simulink model "pid_parallel_sim"  (R2023a)
settings: Solver=VariableStepAuto  StartTime=0.0  StopTime=0.2  MaxStep=Ts  RelTol=1e-3
values from neighbouring files (symbols this model uses):
  fcutD = fp    (= 300)    [pid_ini_parallel.m]
  fcutrollOff = ff    (= 500)    [pid_ini_parallel.m]
  fp = fp_s    (= 300)    [pid_ini_parallel.m]    (also in pid_ini_series.m)
  g_awr = 1.2    [pid_ini_parallel.m]    (also in pid_ini_series.m = 1)
  Kd = -(Ki_s*fp_s - Ki_s*fz_s - 2*pi*Kp_s*fp_s^2 + 2*pi*Kp_s*fp_s*fz_s)/(4*fp_s^2*fz_s*pi^2)    (= 0.176396728594)    [pid_ini_parallel.m]
  Ki = Ki_s    (= 2356.19449019)    [pid_ini_parallel.m]    (also in pid_ini_series.m)
  Kp = (Ki_s*fp_s - Ki_s*fz_s + 2*pi*Kp_s*fp_s*fz_s)/(2*fp_s*fz_s*pi)    (= 42.5)    [pid_ini_parallel.m]    (also in pid_ini_series.m = 25)
  Ts = 50e-6    (= 5e-05)    [pid_ini_parallel.m]    (also in pid_ini_series.m)
  u_max = 5.5    [pid_ini_parallel.m]    (also in pid_ini_series.m)
  u_min = -u_max    (= -5.5)    [pid_ini_parallel.m]    (also in pid_ini_series.m)
  uMax = u_max    (= 5.5)    [pid_ini_parallel.m]
  uMin = u_min    (= -5.5)    [pid_ini_parallel.m]
libraries: cstblocks x8
settings Model: Creator=Michael Peter  LastModifiedBy=Michael Peter

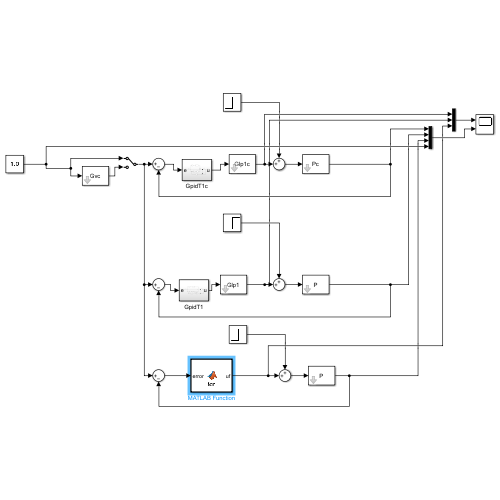
[thumbnail: Simulink's stored preview of the top-level diagram]
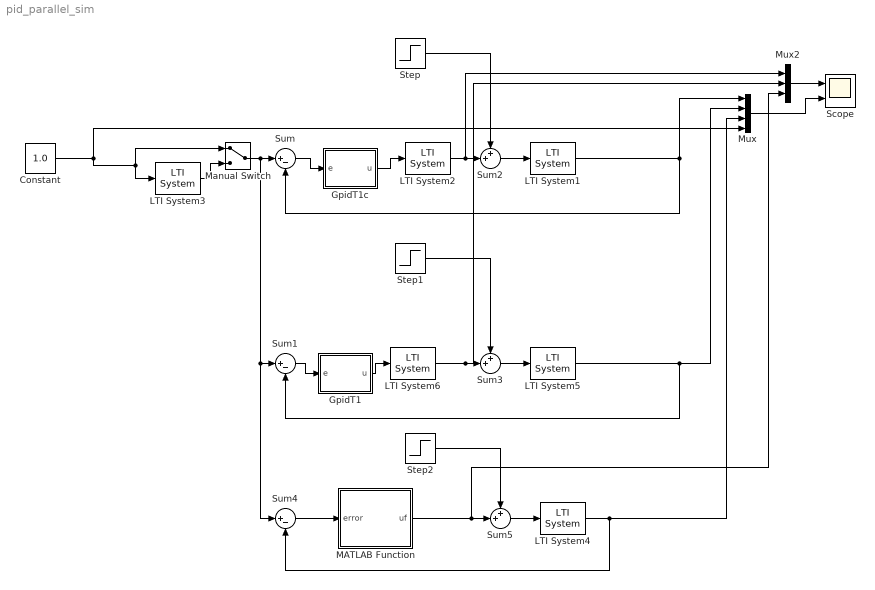
== system pid_parallel_sim ==
  Constant : Constant  Value=1.0
  GpidT1 : Subsystem
  GpidT1c : Subsystem
  LTI System1 : cstblocks/LTI System  sys=Pc  IC=[]
  LTI System2 : cstblocks/LTI System  sys=Glp1c  IC=[]
  LTI System3 : cstblocks/LTI System  sys=Gvc  IC=[]
  LTI System4 : cstblocks/LTI System  sys=P  IC=[]
  LTI System5 : cstblocks/LTI System  sys=P  IC=[]
  LTI System6 : cstblocks/LTI System  sys=Glp1  IC=[]
  MATLAB Function : MATLAB Function  TreatAsAtomicUnit=on
  Manual Switch : ManualSwitch
  Mux : Mux
  Mux2 : Mux  Inputs=3
  Scope : Scope  NumInputPorts=2
  Step : Step  Time=0.12  After=3.5  SampleTime=0
  Step1 : Step  Time=0.12  After=3.5  SampleTime=0
  Step2 : Step  Time=0.12  After=3.5  SampleTime=0
  Sum : Sum  Inputs=|+-
  Sum1 : Sum  Inputs=|+-
  Sum2 : Sum  Inputs=++|
  Sum3 : Sum  Inputs=++|
  Sum4 : Sum  Inputs=|+-
  Sum5 : Sum  Inputs=++|
  wires:
  Sum/1 -> GpidT1c/1(e)
  LTI System1/1 -> Mux/1, Sum/2
  GpidT1c/1(u) -> LTI System2/1
  Sum2/1 -> LTI System1/1
  Mux/1 -> Scope/2
  Step/1 -> Sum2/1
  Manual Switch/1 -> Sum4/1, Sum1/1, Sum/1
  LTI System3/1 -> Manual Switch/2
  Step1/1 -> Sum3/1
  Sum3/1 -> LTI System5/1
  GpidT1/1(u) -> LTI System6/1
  LTI System5/1 -> Mux/2, Sum1/2
  Sum1/1 -> GpidT1/1(e)
  Mux2/1 -> Scope/1
  Sum4/1 -> MATLAB Function/1(error)
  LTI System4/1 -> Mux/3, Sum4/2
  Constant/1 -> Manual Switch/1, LTI System3/1, Mux/4
  Step2/1 -> Sum5/1
  Sum5/1 -> LTI System4/1
  MATLAB Function/1(uf) -> Mux2/3, Sum5/2
  LTI System6/1 -> Mux2/2, Sum3/2
  LTI System2/1 -> Mux2/1, Sum2/2

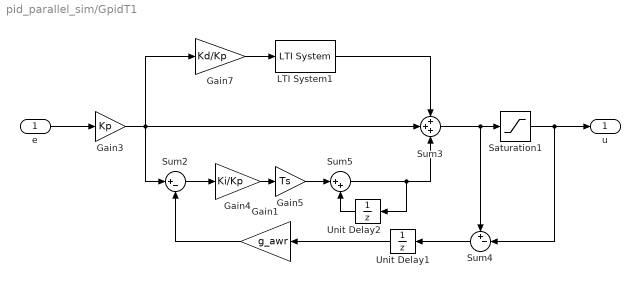
== system pid_parallel_sim/GpidT1 ==
  e : Inport
  Gain1 : Gain  Gain=g_awr
  Gain3 : Gain  Gain=Kp
  Gain4 : Gain  Gain=Ki/Kp
  Gain5 : Gain  Gain=Ts
  Gain7 : Gain  Gain=Kd/Kp
  LTI System1 : cstblocks/LTI System  sys=Gd  IC=[]
  Saturation1 : Saturate  UpperLimit=u_max  LowerLimit=u_min
  Sum2 : Sum  Inputs=|+-
  Sum3 : Sum  Inputs=+++
  Sum4 : Sum  Inputs=+-|
  Sum5 : Sum  Inputs=|++
  Unit Delay1 : UnitDelay  SampleTime=Ts  HasFrameUpgradeWarning=on
  Unit Delay2 : UnitDelay  SampleTime=Ts  HasFrameUpgradeWarning=on
  u : Outport
  wires:
  Gain1/1 -> Sum2/2
  e/1 -> Gain3/1
  Sum5/1 -> Sum3/3, Unit Delay2/1
  Gain5/1 -> Sum5/1
  Gain3/1 -> Gain7/1, Sum3/2, Sum2/1
  Sum2/1 -> Gain4/1
  Gain4/1 -> Gain5/1
  Sum4/1 -> Unit Delay1/1
  Sum3/1 -> Sum4/1, Saturation1/1
  Saturation1/1 -> u/1, Sum4/2
  Unit Delay1/1 -> Gain1/1
  Unit Delay2/1 -> Sum5/2
  Gain7/1 -> LTI System1/1
  LTI System1/1 -> Sum3/1

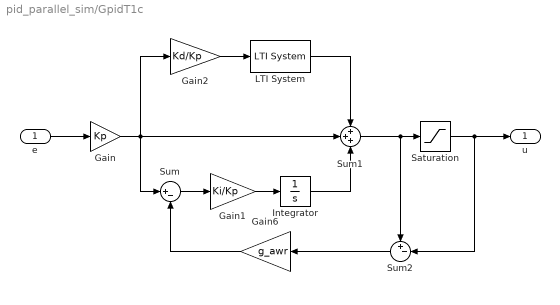
== system pid_parallel_sim/GpidT1c ==
  e : Inport
  Gain : Gain  Gain=Kp
  Gain1 : Gain  Gain=Ki/Kp
  Gain2 : Gain  Gain=Kd/Kp
  Gain6 : Gain  Gain=g_awr
  Integrator : Integrator
  LTI System : cstblocks/LTI System  sys=(2*pi*fp) * tf([1 0], [1 2*pi*fp])  IC=[]
  Saturation : Saturate  UpperLimit=u_max  LowerLimit=u_min
  Sum : Sum  Inputs=|+-
  Sum1 : Sum  Inputs=+++
  Sum2 : Sum  Inputs=+-|
  u : Outport
  wires:
  Saturation/1 -> u/1, Sum2/2
  Sum1/1 -> Sum2/1, Saturation/1
  Gain1/1 -> Integrator/1
  Sum2/1 -> Gain6/1
  Gain/1 -> Sum1/2, Gain2/1, Sum/1
  Sum/1 -> Gain1/1
  e/1 -> Gain/1
  Gain2/1 -> LTI System/1
  Integrator/1 -> Sum1/3
  LTI System/1 -> Sum1/1
  Gain6/1 -> Sum/2

== matlab function pid_parallel_sim/MATLAB Function ==
  settings: updateMethod=DISCRETE  sampleTime=Ts
  data: uf output; Kp parameter; Ki parameter; Kd parameter; fcutD parameter; fcutrollOff parameter; Ts parameter; uMax parameter; uMin parameter; error input
function uf = fcn(Kp, Ki, Kd, fcutD, fcutrollOff, Ts, uMax, uMin, error)

persistent uiPrevious b0_dlpf1 a0_dlpf1 w_dlpf b0_lpf1 a0_lpf1 w_lpf
if isempty(uiPrevious)
    uiPrevious = 0.0;
    % differentiating lowpass 1
    % B = [b0/Ts, -b0/Ts];
    % A = [1, a0];
    b0_dlpf1 = 1.0 - exp(-Ts * 2.0 * pi * fcutD);
    a0_dlpf1 = b0_dlpf1 - 1.0;
    w_dlpf = 0.0;
    % lowpass 1
    % B = [b0, 0];
    % A = [1, a0];
    b0_lpf1 = 1.0 - exp(-Ts * 2.0 * pi * fcutrollOff);
    a0_lpf1 = b0_lpf1 - 1.0;
    w_lpf = 0.0;
end

    % proportional term
    up = Kp * error;

    % constrained integral term
    ui = Ki * error * Ts + uiPrevious;
    if (ui < uMin)
        ui = uMin;
    elseif (ui > uMax)
        ui = uMax;
    end
    uiPrevious = ui;
    
    % derivative term
    def    =  b0_dlpf1 / Ts * error + w_dlpf;
    w_dlpf = -b0_dlpf1 / Ts * error - a0_dlpf1 * def;
    ud = Kd * def;

    % pid sum
    u = up + ui + ud;

    % apply constrained roll off filter
    uf = b0_lpf1 * u + w_lpf;
    if (uf < uMin)
        uf = uMin;
    elseif (uf > uMax)
        uf = uMax;
    end
    w_lpf = - a0_lpf1 * uf;

end
